simulink model "sf_func"  (R2015b)
settings: Solver=ode45  StartTime=0.0  StopTime=100  RelTol=1e-3
libraries: simulink x1
settings Model: Creator=amatsumo  LastModifiedBy=amatsumo
settings DataIOCC: SaveFormat=Array  SignalLoggingSaveFormat=ModelDataLogs
settings OptimizationCC: BlockReduction=off  ConditionallyExecuteInputs=off  ExpressionDepthLimit=2147483647
settings DebuggingCC: UnderspecifiedInitializationDetection=Classic  MergeDetectMultiDrivingBlocksExec=none  SolverPrmCheckMsg=warning  FcnCallInpInsideContextMsg=UseLocalSettings  StateNameClashWarn=warning
settings HardwareCC: ProdBitPerPointer=32  ProdLargestAtomicFloat=None  ProdIntDivRoundTo=Undefined  ProdEndianess=Unspecified  ProdWordSize=32  ProdHWDeviceType=32-bit Generic
settings GRTTargetCC: GeneratePreprocessorConditionals=Disable all  CombineOutputUpdateFcns=off  GRTInterface=on
settings ConfigComp: CovModelRefEnable=Off  CovSFcnEnable=off

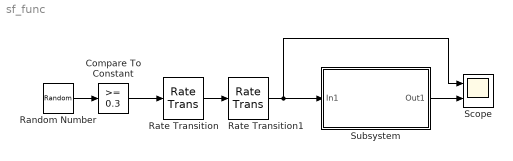
== system sf_func ==
  Compare To Constant : simulink/Logic and Bit Operations/Compare To Constant  relop=>=  const=0.3  OutDataTypeStr=boolean
  Random Number : RandomNumber  SampleTime=0.01
  Rate Transition : RateTransition  OutPortSampleTime=0.1
  Rate Transition1 : RateTransition  OutPortSampleTime=1
  Scope : Scope  NumInputPorts=2
  Subsystem : Subsystem
  wires:
  Compare To Constant/1 -> Rate Transition/1
  Subsystem/1(Out1) -> Scope/2
  Random Number/1 -> Compare To Constant/1
  Rate Transition/1 -> Rate Transition1/1
  Rate Transition1/1 -> Scope/1, Subsystem/1(In1)

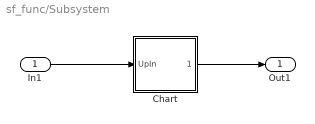
== system sf_func/Subsystem ==
  In1 : Inport
  Chart : Stateflow chart  TreatAsAtomicUnit=on
  Out1 : Outport
  wires:
  In1/1 -> Chart/1(UpIn)
  Chart/1(DataOut) -> Out1/1

== stateflow chart sf_func/Subsystem/Chart ==
  settings: stateMachineType=MEALY_MACHINE  executeAtInitialization=1  initializeOutput=1
  state Data = inc_data(Up,tmp) [function]
    (default) -> (junction 2)
    (junction 2) -> (junction 3) [order 1] : [Up == 1]
        | {Data=tmp+1}
    (junction 3) -> (junction 26)
    (junction 2) -> (junction 4) [order 2]
    (junction 26) -> (junction 4) [order 1] : [Data >= 10]
        | { Data = 0;}
    (junction 26) -> (junction 28) [order 2]
    (junction 4) -> (junction 11)
  (default) -> (junction 21) : {temp = inc_data(UpIn,temp);
      | DataOut = temp;}
  data: Up function_input boolean; Data function_output int8; tmp function_input int8; DataOut output int8; UpIn input boolean; temp local int8
